simulink model "func1_d"  (R2019b)
settings: Solver=VariableStepAuto  StartTime=0.0  StopTime=10.0  RelTol=1e-3  EnableMultiTasking=on
libraries: ModelComposer x2, fixedpoint_complex_1_lib x1
settings Model: Creator=abehbood  LastModifiedBy=abehbood
settings DataIOCC: ReturnWorkspaceOutputs=off
settings OptimizationCC: LifeSpan=inf
settings DebuggingCC: SFUnexpectedBacktrackingDiag=warning  SFNoUnconditionalDefaultTransitionDiag=warning  ArithmeticOperatorsInVariantConditions=warning
settings SFSimCC: SimUseLocalCustomCode=off  CustomCodeUndefinedFunction=UseInterfaceOnly
settings RTWCC: RTWUseLocalCustomCode=off
settings CodeAppCC: StateflowObjectComments=on
settings GRTTargetCC: TargetLangStandard=C89/C90 (ANSI)
settings ConfigComp: CovMetricSettings=dw  CovHtmlReporting=on  CovSaveCumulativeToWorkspaceVar=on  CovSaveSingleToWorkspaceVar=on  CovExternalEMLEnable=off

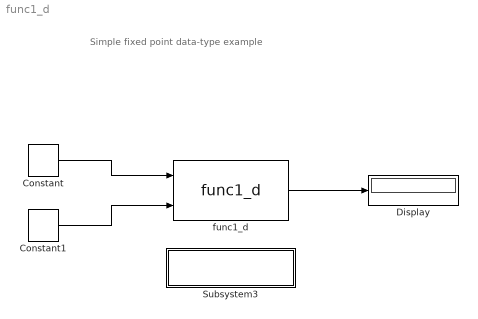
== system func1_d ==
  note: Simple fixed point data-type example
  Constant : ModelComposer/Constant  Value=20  VectorParams1D=off  SampleTime=1.0  OutDataType=fixed  TypeExp=''  Signedness=Signed  WordLength=16  FractionalLength=5  RoundingMode=Truncation to minus infinity  OverflowMode=Wrap around
  Constant1 : ModelComposer/Constant  Value=40  VectorParams1D=off  SampleTime=1.0  OutDataType=fixed  TypeExp=''  Signedness=Signed  WordLength=16  FractionalLength=5  RoundingMode=Truncation to minus infinity  OverflowMode=Wrap around
  Display : Display
  Subsystem3 : Subsystem
      settings: OpenFcn=xmcOpenFileEx
      mask Display: disp(sprintf('Double Click to open\nthe main header file'))
  func1_d : fixedpoint_complex_1_lib/func1_d  LibraryFunction=func1_d  IncludeFiles={'func1_d.h'}  SourceFiles={}  IncludeDirectories={}  TemplateParams={' '}  FunctionParamTypes={xmcDataType('void'); xmcDataType('const ap_fixed<16, 11>'); xmcDataType('const ap_fixed<16, 11>'); xmcDataType('ap_fixed<17, 11> &')}  FunctionParamPassbys={0.000000000000000000e+00; 0.000000000000000000e+00; 0.000000000000000000e+00; 1.000000000000000000e+00}  FunctionParamDimensions={'1'; '1'; '1'; '1'}  FunctionParamNames={'return'; 'in1'; 'in2'; 'out'}  FunctionParamDir={0.000000000000000000e+00; 1.000000000000000000e+00; 1.000000000000000000e+00; 2.000000000000000000e+00}  FunctionParamSupportsStreaming={false; false; false; false}  BufferDepth={'0'}  FunctionParamValues={'0'; '0'; '0'; '0'}  ThroughputFactors={''}
  wires:
  Constant/1 -> func1_d/1
  Constant1/1 -> func1_d/2
  func1_d/1 -> Display/1

== system func1_d/Subsystem3 ==
